simulink model "mr_cpm_test2"  (R2014b)
settings: Solver=ode45  StartTime=0.0  StopTime=1  RelTol=1e-3
libraries: commdigbbndpm3 x2, commrandsrc2 x2, commdigbbndcpm2 x1, commsink2 x1, dspmlti4 x1, commchan3 x1
settings Model: Creator=joel2  LastModifiedBy=joel2

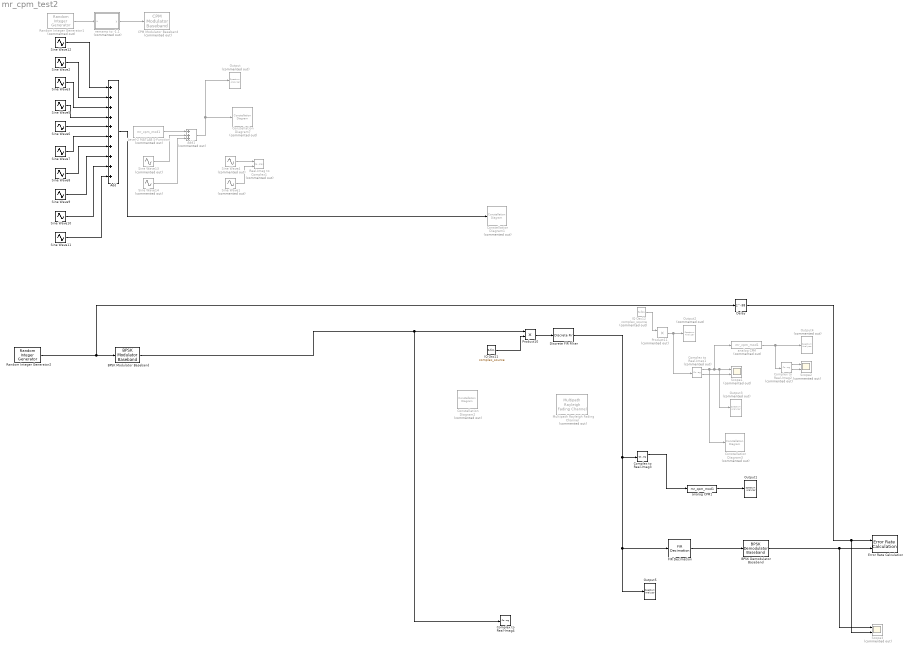
== system mr_cpm_test2 ==
  Add : Sum  Inputs=++++++++++
  Add1 : Sum  Commented=on  Inputs=+++
  BPSK Demodulator Baseband : commdigbbndpm3/BPSK Demodulator Baseband  Ph=0  DecType=Hard decision  VarSource=Dialog  Variance=1  outDtype=Inherit via internal rule  derotateFactorWordLen=16
  BPSK Modulator Baseband : commdigbbndpm3/BPSK Modulator Baseband  Ph=0  outDtype=double  outWordLen=16  outUDDataType=sfix(16)  outFracLenMode=Best precision  outFracLen=15
  CPM Modulator Baseband : commdigbbndcpm2/CPM Modulator Baseband  Commented=on  Mnum=4  inputType=Integer  mappingType=Binary  modIdx=0.5  pulseShape=Rectangular  BT=0.3  mainLobePulseLength=1  rollOff=0.2  pulseLength=1  preHistory=1  phaseOffset=0  samplesPerSymbol=8  RateOptions=Enforce single-rate processing  outDataType=double
  Complex to Real-Imag1 : ComplexToRealImag  Commented=on
  Complex to Real-Imag2 : ComplexToRealImag  Commented=on
  Complex to Real-Imag3 : ComplexToRealImag
  Complex to Real-Imag4 : ComplexToRealImag
  Constellation Diagram{1..3,7} (4 alike) : ConstellationDiagram  Commented=on
  Delay : Delay  DelayLength=38  InitialCondition=0
  Discrete FIR Filter : DiscreteFir  Coefficients=0.35*sinc(0.35*(-100:100))
  Error Rate Calculation : commsink2/Error Rate Calculation  N=0  st_delay=0  cp_mode=Entire frame  subframe=[]  PMode=Workspace  WsName=ErrorVec  RsMode2=off  stop=off  numErr=100  maxBits=1e6
  FIR Decimation : dspmlti4/FIR Decimation  h=fir1(100,0.35)  D=4  filtStruct=Direct form  framing=Allow multirate processing  inputOffset=0  outputBufInitCond=0  firstCoeffDataTypeStr=Inherit: Same word length as input  firstCoeffLastDataTypeStr=Inherit: Same word length as input  firstCoeffMin=[]  firstCoeffMax=[]  outputDataTypeStr=Inherit: Same as accumulator  outputLastDataTypeStr=Inherit: Same as accumulator  outputMin=[]  outputMax=[]  roundingMode=Floor  overflowMode=off  FilterSource=Specify via dialog  FilterObject=Hm_firdecim
      settings: allowOverrides=off
  IQ Osc11 : M-S-Function  FunctionName=complex_source  Parameters=Freq, SampleTime  mask{Freq=0, SampleTime=1/40000}
      mask prompts: Freq "Frequency (rads):"; SampleTime "Sample Time (s):"
      mask Display: image('complex_source2.svg')
  IQ Osc12 : M-S-Function  Commented=on  FunctionName=complex_source  Parameters=Freq, SampleTime  mask{Freq=5000*2*pi, SampleTime=1/40000}
      mask prompts: Freq "Frequency (rads):"; SampleTime "Sample Time (s):"
      mask Display: image('complex_source2.svg')
  Level-2 MATLAB S-Function : M-S-Function  Commented=on  FunctionName=mr_cpm_mod1
  Multipath Rayleigh Fading Channel : commchan3/Multipath Rayleigh Fading Channel  Commented=on  maxDopplerShift=40  spectrumType=Jakes  sigmaGaussian=1/sqrt(2)  coeffRounded=[1 -1.72 0.785]  freqMinMaxRJakes=[0 1]  freqMinMaxAJakes=[0 1]  sigmaGaussian1=1/sqrt(2)  sigmaGaussian2=1/sqrt(2)  centerFreqGaussian1=0.0  centerFreqGaussian2=0.0  gainGaussian1=0.5  gainGaussian2=0.5  coeffBell=9  dopplerSpectrum=doppler.jakes  pathDelays=[0 2e-6]  avgPathGaindB=[0 -3]  normalizePathGains=on  seed=73  enableProbe=0  openVisAtStart=off  outPathGains=off  outDelay=off
  Output{,2..4} (4 alike) : SpectrumAnalyzer  Commented=on
  Output1 : SpectrumAnalyzer
  Output5 : SpectrumAnalyzer
  Product10 : Product
  Product11 : Product  Commented=on
  Random Integer Generator1 : commrandsrc2/Random Integer Generator  Commented=on  mul=2  seed=42  Ts=1/(10000)  frameBased=off  sampPerFrame=1024  orient=off  outDataType=double
  Random Integer Generator2 : commrandsrc2/Random Integer Generator  mul=2  seed=42  Ts=1/(10000)  frameBased=off  sampPerFrame=1  orient=off  outDataType=double
  Real-Imag to Complex1 : RealImagToComplex  Commented=on
  Scope1 : Scope  Commented=on  NumInputPorts=2
      settings: YMin=-5~-5  YMax=5~5
  Scope2 : Scope  Commented=on  NumInputPorts=2
      settings: YMin=-5~-5  YMax=5~5  SaveName=ScopeData2
  Scope3 : Scope  Commented=on  NumInputPorts=2
      settings: YMin=-5~-5  YMax=5~5  MaxDataPoints=20000
  Sine Wave1 : Sin  Commented=on  Frequency=12.801*2*pi*1000  Phase=-pi/2  SampleTime=1/128000
  Sine Wave10 : Sin  Amplitude=0.1  Frequency=98*2*pi  SampleTime=1/128000
  Sine Wave11 : Sin  Amplitude=0.1  Frequency=99*2*pi  SampleTime=1/128000
  Sine Wave12 : Sin  Amplitude=0.1  Frequency=100*2*pi  SampleTime=1/128000
  Sine Wave13 : Sin  Commented=on  Frequency=10*2*pi  SampleTime=1/128000
  Sine Wave14 : Sin  Commented=on  Frequency=20*2*pi  SampleTime=1/128000
  Sine Wave2 : Sin  Amplitude=0.1  Frequency=91*2*pi  SampleTime=1/128000
  Sine Wave3 : Sin  Amplitude=0.1  Frequency=92*2*pi  SampleTime=1/128000
  Sine Wave4 : Sin  Commented=on  Frequency=12.801*2*pi*1000  SampleTime=1/128000
  Sine Wave5 : Sin  Amplitude=0.1  Frequency=93*2*pi  SampleTime=1/128000
  Sine Wave6 : Sin  Amplitude=0.1  Frequency=94*2*pi  SampleTime=1/128000
  Sine Wave7 : Sin  Amplitude=0.1  Frequency=95*2*pi  SampleTime=1/128000
  Sine Wave8 : Sin  Amplitude=0.1  Frequency=96*2*pi  SampleTime=1/128000
  Sine Wave9 : Sin  Amplitude=0.1  Frequency=97*2*pi  SampleTime=1/128000
  analog CPM : M-S-Function  Commented=on  FunctionName=mr_cpm_mod1
      mask Display: image('mr_cpm_mod1.svg');
  analog CPM1 : M-S-Function  FunctionName=mr_cpm_mod1
      mask Display: image('mr_cpm_mod1.svg');
  remamp to -1,1 : MATLAB Function  Commented=on  TreatAsAtomicUnit=on
  wires:
  Sine Wave4/1 -> Real-Imag to Complex1/1
  Sine Wave1/1 -> Real-Imag to Complex1/2
  Random Integer Generator1/1 -> remamp to -1,1/1(u)
  remamp to -1,1/1(y) -> CPM Modulator Baseband/1
  Sine Wave12/1 -> Add/1
  Sine Wave2/1 -> Add/2
  Sine Wave3/1 -> Add/3
  Sine Wave5/1 -> Add/4
  Sine Wave6/1 -> Add/5
  Sine Wave7/1 -> Add/6
  Sine Wave8/1 -> Add/7
  Sine Wave9/1 -> Add/8
  Sine Wave10/1 -> Add/9
  Sine Wave11/1 -> Add/10
  Level-2 MATLAB S-Function/1 -> Add1/1
  Sine Wave13/1 -> Add1/2
  Add1/1 -> Constellation Diagram7/1, Output/1
  Sine Wave14/1 -> Add1/3
  IQ Osc11/1 -> Product10/2
  IQ Osc12/1 -> Product11/1
  Product11/1 -> Complex to Real-Imag1/1, Output2/1
  Complex to Real-Imag1/1 -> Constellation Diagram3/1, analog CPM/1, Output3/1, Scope1/1
  Complex to Real-Imag1/2 -> Scope1/2
  analog CPM/1 -> Complex to Real-Imag2/1, Output4/1
  Complex to Real-Imag2/1 -> Scope2/1
  Complex to Real-Imag2/2 -> Scope2/2
  Add/1 -> Constellation Diagram1/1
  BPSK Modulator Baseband/1 -> Complex to Real-Imag4/1, Product10/1
  FIR Decimation/1 -> BPSK Demodulator Baseband/1
  Product10/1 -> Discrete FIR Filter/1
  BPSK Demodulator Baseband/1 -> Error Rate Calculation/2, Scope3/1
  Random Integer Generator2/1 -> Delay/1, BPSK Modulator Baseband/1
  Delay/1 -> Error Rate Calculation/1, Scope3/2
  Discrete FIR Filter/1 -> Complex to Real-Imag3/1, Output5/1, FIR Decimation/1
  analog CPM1/1 -> Output1/1
  Complex to Real-Imag3/1 -> analog CPM1/1

== matlab function mr_cpm_test2/remamp to -1,1 ==
  data: u input; y output
function y = fcn(u)
%#codegen

y = (u*2)-1;
